simulink model "bm99mld"  (Simulink 5.0)
settings: Solver=ode45  StartTime=0.0  StopTime=Tstop  RelTol=1e-3
values from neighbouring files (symbols this model uses):
  C = hybcon(S,Q,N,limits,refs)    [binary_inputs_sim.m]    (also in bm99benchmark.m; bm99norm2.m; bm99sim.m; exp2mld_mimo.m = lincon(model,'track',cost,interval,limits))
libraries: hyblib x2
settings Model: LastModifiedBy=Alberto Bemporad

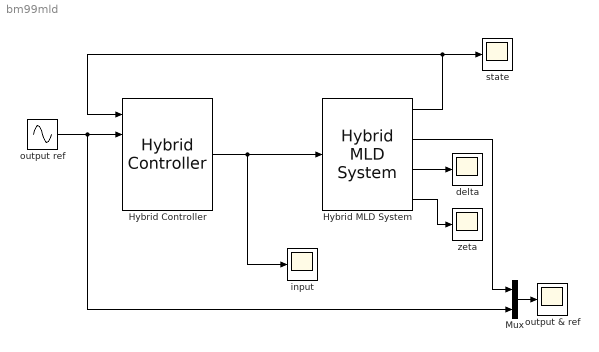
== system bm99mld ==
  Hybrid Controller : hyblib/Hybrid Controller  C=C  S=S  tilim=Inf
  Hybrid MLD System : hyblib/Hybrid MLD System  S=S  x0init=x0
  Mux : Mux  Inputs=2
  delta : Scope
  input : Scope
      settings: TimeRange=100  YMin=-1  YMax=0.4  SaveName=ScopeData2
  output & ref : Scope
      settings: TimeRange=100  YMin=-1  YMax=1  SaveName=ScopeData4
  output ref : Sin  Frequency=1/8  SampleTime=0
  state : Scope
      settings: SaveName=ScopeData3
  zeta : Scope
  wires:
  Hybrid Controller/1 -> Hybrid MLD System/1, input/1
  output ref/1 -> Hybrid Controller/2, Mux/2
  Mux/1 -> output & ref/1
  Hybrid MLD System/1 -> state/1, Hybrid Controller/1
  Hybrid MLD System/2 -> Mux/1
  Hybrid MLD System/3 -> delta/1
  Hybrid MLD System/4 -> zeta/1
